simulink model "minus1"  (R2018a)
settings: Solver=VariableStepAuto  StartTime=0.0  StopTime=10.0  RelTol=1e-3
settings Model: Creator=berke  LastModifiedBy=berke

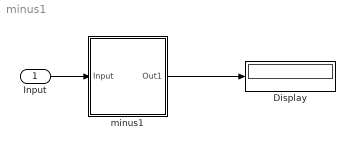
== system minus1 ==
  Input : Inport  OutDataTypeStr=fixdt(1,32,15)  SampleTime=0.1
  Display : Display
  minus1 : Subsystem
  wires:
  minus1/1(Out1) -> Display/1
  Input/1 -> minus1/1(Input)

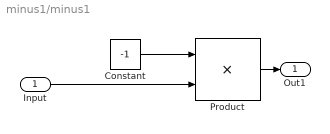
== system minus1/minus1 ==
  Input : Inport
  Constant : Constant  Value=-1  OutMin=-1  OutMax=-1  OutDataTypeStr=fixdt(1,2,1)  SampleTime=0.1
  Product : Product
  Out1 : Outport
  wires:
  Product/1 -> Out1/1
  Constant/1 -> Product/1
  Input/1 -> Product/2
